simulink model "Model2"  (R2014b)
settings: Solver=ode45  StartTime=0.0  StopTime=10.0  RelTol=1e-3
values from neighbouring files (symbols this model uses):
  dt = 9.2e6    (= 9200000)    [Parameters.m]
  Jpp = 1e6    (= 1000000)    [Parameters.m]
  Jt = 1.56e8    (= 156000000)    [Parameters.m]
  kt = 2.3e9    (= 2300000000)    [Parameters.m]
  phs = 40    [Parameters.m]
  Q = G    (= 7.5)    [Parameters.m]
  Tpull = 11.9e6    (= 11900000)    [Parameters.m]
libraries: re_lib x1, powerlib x1
settings Model: Creator=Eduardo Montilva  LastModifiedBy=Eduardo Montilva
settings DebuggingCC: UnconnectedInputMsg=none  UnconnectedOutputMsg=none  UnconnectedLineMsg=none

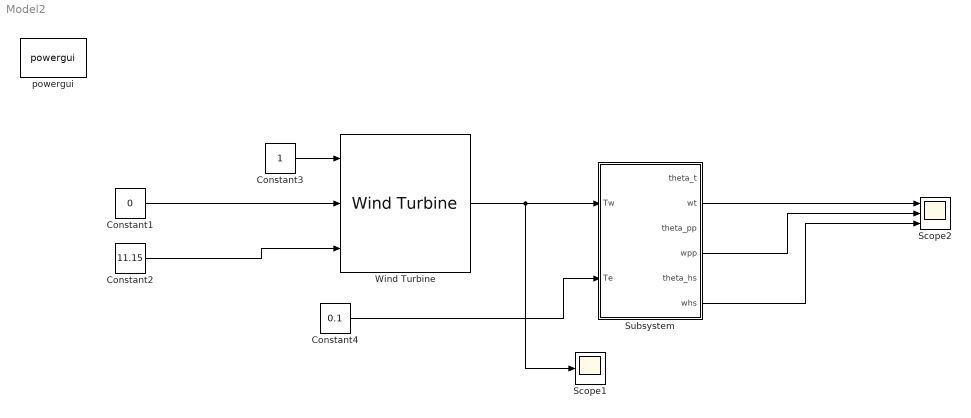
== system Model2 ==
  Constant1 : Constant  Value=0
  Constant2 : Constant  Value=11.15
  Constant3 : Constant
  Constant4 : Constant  Value=0.1
  Scope1 : Scope
      settings: YMin=-1.09999  YMax=-0.89999
  Scope2 : Scope  NumInputPorts=3
      settings: YMin=-4.5e-08~-5e-08~-0.0008  YMax=0~3e-08~0.0008
  Subsystem : Subsystem
  Wind Turbine : re_lib/Wind Generation/Wind Turbine  Pnom=1.5e6  Pelec_base=1.5e6/0.9  wind_base=12  P_wind_base=0.73  speed_nom=1.2  pitch_angle=0  DisplayTurbChar=off  c1_c6="[0.51763          116          0.4            5           21     0.006795]"  cp_nom=0.48  lambda_nom=8.1
  powergui : powerlib/powergui  Priority=1  SimulationMode=Phasor  SolverType=Tustin/Backward Euler (TBE)  SampleTime=50e-6  frequency=60  SPID=off  DisableSnubberDevices=off  DisableRonSwitches=off  DisableVfSwitches=off  SwTol=0  DisplayEquations=off  Interpol=off  methode=off  Ts=100  frequencyindice=60  Pbase=100e6  ErrMax=1e-4  Iterations=50  UnitsV=kV  UnitsW=MW  FunctionMessages=off  echomessages=off  HookPort=off  EnableUseOfTLC=off  x0status=blocks  RestoreLinks=warning  ResistiveCurrentMeasurement=off  Frange=[0:2:500]  Ylog=off  Xlog=on  ShowGrid=off  save=off  variable=ZData  structure=0  ZoomFFT=off  StartTime=0.0  cycles=1  DisplayStyle=1  fundamental=60  FreqAxis=off  MaxFrequency=1000  frequencyindicesteady=1  RmsSteady=1  display=off
  wires:
  Constant2/1 -> Wind Turbine/3
  Constant1/1 -> Wind Turbine/2
  Constant3/1 -> Wind Turbine/1
  Wind Turbine/1 -> Scope1/1, Subsystem/1(Tw)
  Subsystem/2(wt) -> Scope2/1
  Subsystem/4(wpp) -> Scope2/2
  Subsystem/6(whs) -> Scope2/3
  Constant4/1 -> Subsystem/2(Te)

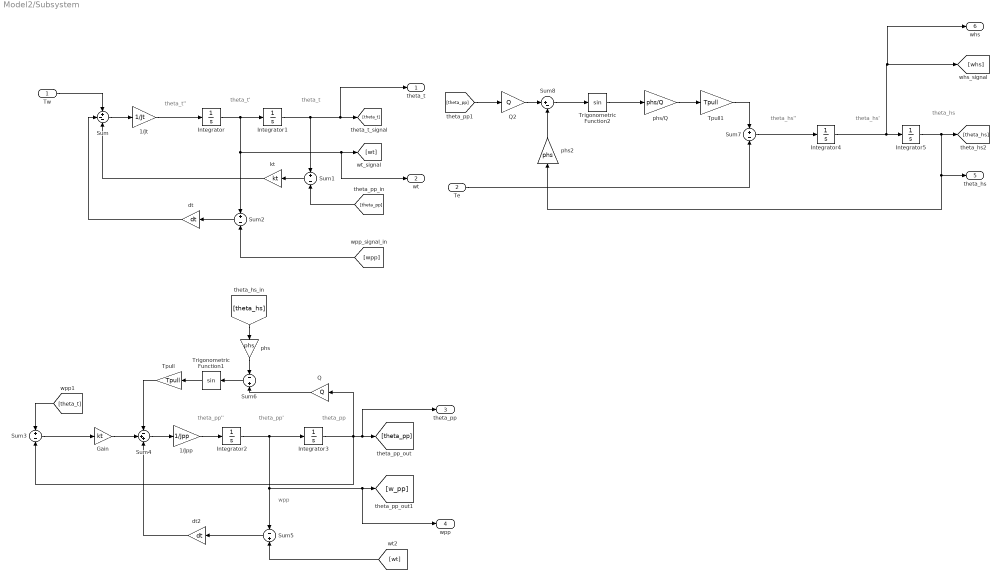
== system Model2/Subsystem ==
  note: theta_hs
  note: theta_hs'
  note: theta_hs''
  note: theta_pp
  note: wpp
  note: theta_pp'
  note: theta_pp''
  note: theta_t
  note: theta_t'
  note: theta_t''
  Tw : Inport
  Te : Inport  Port=2
  1/Jpp : Gain  Gain=1/Jpp
  1/Jt : Gain  Gain=1/Jt
  Gain : Gain  Gain=kt
  Integrator{,1..5} (6 alike) : Integrator
  Q : Gain  Gain=Q
  Q2 : Gain  Gain=Q
  Sum : Sum  Inputs=+--
  Sum1 : Sum  Inputs=+-
  Sum2 : Sum  Inputs=+-
  Sum3 : Sum  Inputs=+|-
  Sum4 : Sum  Inputs=-++
  Sum5 : Sum  Inputs=-+
  Sum6 : Sum  Inputs=-|+
  Sum7 : Sum  Inputs=+-
  Sum8 : Sum  Inputs=|+-
  Tpull : Gain  Gain=Tpull
  Tpull1 : Gain  Gain=Tpull
  Trigonometric Function1 : Trigonometry
  Trigonometric Function2 : Trigonometry
  dt : Gain  Gain=dt
  dt2 : Gain  Gain=dt
  kt : Gain  Gain=kt
  phs : Gain  Gain=phs
  phs/Q : Gain  Gain=phs/Q
  phs2 : Gain  Gain=phs
  theta_t : Outport
  wt : Outport  Port=2
  theta_pp : Outport  Port=3
  wpp : Outport  Port=4
  theta_hs : Outport  Port=5
  whs : Outport  Port=6
  wires:
  Trigonometric Function2/1 -> phs/Q/1
  Integrator5/1 -> theta_hs/1, phs2/1, [theta_hs]
  Sum7/1 -> Integrator4/1
  Integrator4/1 -> whs/1, [whs], Integrator5/1
  1/Jpp/1 -> Integrator2/1
  Integrator3/1 -> Sum3/2, Q/1, theta_pp/1, [theta_pp]
  Integrator2/1 -> wpp/1, [w_pp], Sum5/1, Integrator3/1
  Sum5/1 -> dt2/1
  Q/1 -> Sum6/2
  Sum1/1 -> kt/1
  [theta_hs] -> phs/1
  phs/1 -> Sum6/1
  kt/1 -> Sum/3
  1/Jt/1 -> Integrator/1
  Tw/1 -> Sum/1
  [wpp] -> Sum2/2
  dt2/1 -> Sum4/3
  Sum6/1 -> Trigonometric Function1/1
  Gain/1 -> Sum4/2
  Sum/1 -> 1/Jt/1
  Integrator1/1 -> theta_t/1, [theta_t], Sum1/1
  [theta_pp] -> Sum1/2
  Sum2/1 -> dt/1
  Sum4/1 -> 1/Jpp/1
  Integrator/1 -> Sum2/1, wt/1, [wt], Integrator1/1
  dt/1 -> Sum/2
  Sum3/1 -> Gain/1
  [theta_t] -> Sum3/1
  [theta_pp] -> Q2/1
  phs2/1 -> Sum8/2
  Sum8/1 -> Trigonometric Function2/1
  Tpull/1 -> Sum4/1
  Trigonometric Function1/1 -> Tpull/1
  phs/Q/1 -> Tpull1/1
  [wt] -> Sum5/2
  Te/1 -> Sum7/2
  Q2/1 -> Sum8/1
  Tpull1/1 -> Sum7/1
